simulink model "validation"  (Simulink 9.3)
settings: Solver=VariableStepAuto  StartTime=0  StopTime=25  FixedStep=0.02  RelTol=1e-3
libraries: Solver_SF x1
settings Model: Creator=cy  LastModifiedBy=cy
settings DataIOCC: SaveFormat=Dataset  SignalLoggingSaveFormat=Dataset  ReturnWorkspaceOutputs=on
settings OptimizationCC: LifeSpan=auto
settings DebuggingCC: UnderspecifiedInitializationDetection=Simplified  MergeDetectMultiDrivingBlocksExec=error  FcnCallInpInsideContextMsg=error  SFUnexpectedBacktrackingDiag=error  SFNoUnconditionalDefaultTransitionDiag=error  SFExecutionAtInitializationDiag=warning  ArithmeticOperatorsInVariantConditions=error
settings HardwareCC: ProdBitPerPointer=64  ProdBitPerSizeT=64  ProdBitPerPtrDiffT=64  ProdLargestAtomicFloat=Float  ProdIntDivRoundTo=Zero  ProdEndianess=LittleEndian  ProdWordSize=64  ProdHWDeviceType=Intel->x86-64 (Windows64)
settings ModelReferenceCC: PropagateSignalLabelsOutOfModel=on
settings SFSimCC: SimUseLocalCustomCode=on
settings RTWCC: RTWUseLocalCustomCode=on
settings CodeAppCC: StateflowObjectComments=off
settings GRTTargetCC: TargetLangStandard=C99 (ISO)  CombineOutputUpdateFcns=on  GRTInterface=off
settings ConfigComp: CovMetricSettings=dwe  CovHtmlReporting=off  CovSaveCumulativeToWorkspaceVar=off  CovSaveSingleToWorkspaceVar=off  CovExternalEMLEnable=on

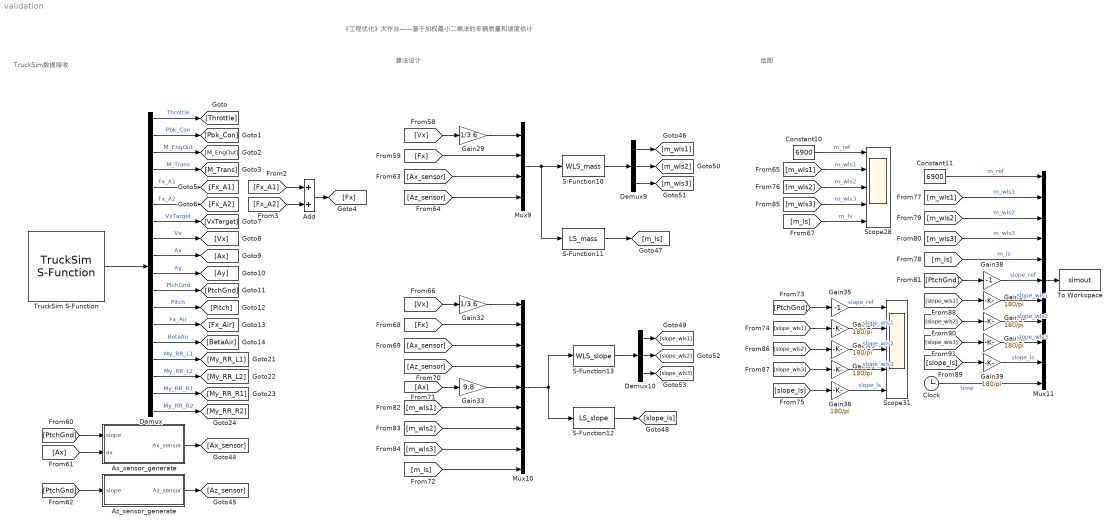
== system validation ==
  note: 《工程优化》大作业——基于加权最小二乘法的车辆质量和坡度估计
  note: TruckSim数据接收
  note: 绘图
  note: 算法设计
  Add : Sum
  Ax_sensor_generate : MATLAB Function  TreatAsAtomicUnit=on
  Az_sensor_generate : MATLAB Function  TreatAsAtomicUnit=on
  Clock : Clock
  Constant10 : Constant  Value=6900
  Constant11 : Constant  Value=6900
  Demux : Demux  Outputs=18
  Demux10 : Demux  Outputs=3
  Demux9 : Demux  Outputs=3
  Gain29 : Gain  Gain=1/3.6
  Gain32 : Gain  Gain=1/3.6
  Gain33 : Gain  Gain=9.8
  Gain{34,36..37,39..43} (8 alike) : Gain  Gain=180/pi
  Gain35 : Gain  Gain=-1
  Gain38 : Gain  Gain=-1
  Mux10 : Mux  Inputs=9
  Mux11 : Mux  Inputs=11
  Mux9 : Mux
  S-Function10 : S-Function  FunctionName=WLS_mass  SFunctionDeploymentMode=off  EnableBusSupport=off
  S-Function11 : S-Function  FunctionName=LS_mass  SFunctionDeploymentMode=off  EnableBusSupport=off
  S-Function12 : S-Function  FunctionName=LS_slope  SFunctionDeploymentMode=off  EnableBusSupport=off
  S-Function13 : S-Function  FunctionName=WLS_slope  SFunctionDeploymentMode=off  EnableBusSupport=off
  Scope28 : Scope  NumInputPorts=5
  Scope31 : Scope  NumInputPorts=5
  To Workspace : ToWorkspace  VariableName=simout  SampleTime=0.02
  TruckSim S-Function : Solver_SF/TruckSim S-Function  Priority=1  SIMFILE=simfile.sim
  wires:
  TruckSim S-Function/1 -> Demux/1
  Demux/13 -> [Fx_Air]  "Fx_Air"
  Demux/14 -> [BetaAir]  "BetaAir"
  Demux/11 -> [PtchGnd]  "PtchGnd"
  Demux/12 -> [Pitch]  "Pitch"
  Demux/4 -> [M_Trans]  "M_Trans"
  Demux/3 -> [M_EngOut]  "M_EngOut"
  Demux/5 -> [Fx_A1]  "Fx_A1"
  Demux/6 -> [Fx_A2]  "Fx_A2"
  Demux/8 -> [Vx]  "Vx"
  Demux/2 -> [Pbk_Con]  "Pbk_Con"
  Demux/1 -> [Throttle]  "Throttle"
  Demux/9 -> [Ax]  "Ax"
  Demux/7 -> [VxTarget]  "VxTarget"
  Demux/10 -> [Ay]  "Ay"
  [Fx_A2] -> Add/2
  [Fx_A1] -> Add/1
  Add/1 -> [Fx]
  Demux/15 -> [My_RR_L1]  "My_RR_L1"
  Demux/16 -> [My_RR_L2]  "My_RR_L2"
  Demux/17 -> [My_RR_R1]  "My_RR_R1"
  Demux/18 -> [My_RR_R2]  "My_RR_R2"
  [Vx] -> Gain29/1
  [Fx] -> Mux9/2
  Gain29/1 -> Mux9/1
  [PtchGnd] -> Ax_sensor_generate/1(slope)
  [Ax] -> Ax_sensor_generate/2(ax)
  Ax_sensor_generate/1(Ax_sensor) -> [Ax_sensor]
  [PtchGnd] -> Az_sensor_generate/1(slope)
  Az_sensor_generate/1(Az_sensor) -> [Az_sensor]
  Mux9/1 -> S-Function10/1, S-Function11/1
  [Ax_sensor] -> Mux9/3
  [Az_sensor] -> Mux9/4
  S-Function10/1 -> Demux9/1
  Constant10/1 -> Scope28/1  "m_ref"
  [m_wls1] -> Scope28/2  "m_wls1"
  S-Function11/1 -> [m_ls]
  [Az_sensor] -> Mux10/4
  Gain32/1 -> Mux10/1
  [Ax_sensor] -> Mux10/3
  [Vx] -> Gain32/1
  Mux10/1 -> S-Function13/1, S-Function12/1
  [Fx] -> Mux10/2
  [Ax] -> Gain33/1
  Gain33/1 -> Mux10/5
  [m_ls] -> Mux10/9
  S-Function12/1 -> [slope_ls]
  Gain34/1 -> Scope31/2  "slope_wls1"
  [PtchGnd] -> Gain35/1
  [slope_wls1] -> Gain34/1
  Gain35/1 -> Scope31/1  "slope_ref"
  [m_ls] -> Scope28/5  "m_ls"
  S-Function13/1 -> Demux10/1
  [slope_ls] -> Gain36/1
  Gain36/1 -> Scope31/5  "slope_ls"
  [m_wls1] -> Mux10/6
  Mux11/1 -> To Workspace/1
  Clock/1 -> Mux11/11  "time"
  Demux9/1 -> [m_wls1]
  Demux9/3 -> [m_wls3]
  Demux9/2 -> [m_wls2]
  [m_wls2] -> Mux10/7
  [m_wls3] -> Mux10/8
  [m_wls3] -> Scope28/4  "m_wls3"
  [m_wls2] -> Scope28/3  "m_wls2"
  Demux10/1 -> [slope_wls1]
  Demux10/3 -> [slope_wls3]
  Demux10/2 -> [slope_wls2]
  [slope_wls2] -> Gain40/1
  Gain40/1 -> Scope31/3  "slope_wls2"
  [slope_wls3] -> Gain41/1
  Gain41/1 -> Scope31/4  "slope_wls3"
  [m_wls1] -> Mux11/2  "m_wls1"
  [m_wls3] -> Mux11/4  "m_wls3"
  [m_wls2] -> Mux11/3  "m_wls2"
  Constant11/1 -> Mux11/1  "m_ref"
  [m_ls] -> Mux11/5  "m_ls"
  [slope_ls] -> Gain39/1
  Gain37/1 -> Mux11/7  "slope_wls1"
  [slope_wls3] -> Gain43/1
  [slope_wls2] -> Gain42/1
  Gain43/1 -> Mux11/9  "slope_wls3"
  Gain38/1 -> Mux11/6  "slope_ref"
  [PtchGnd] -> Gain38/1
  Gain39/1 -> Mux11/10  "slope_ls"
  Gain42/1 -> Mux11/8  "slope_wls2"
  [slope_wls1] -> Gain37/1

== matlab function Az_sensor_generate ==
  data: slope input double; Az_sensor output double
function Az_sensor = fcn(slope)
slope = slope * pi /180;

Az_sensor = 9.8 * cos(slope);

== matlab function Ax_sensor_generate ==
  data: slope input double; Ax_sensor output double; ax input double
function Ax_sensor = fcn(slope, ax)
slope = slope * pi /180;
ax = ax * 9.8;

Ax_sensor = 9.8 * sin(-slope) + ax;
